simulink model "SF018A_EotProtn"  (R2013b)
settings: Solver=FixedStepDiscrete  SolverMode=SingleTasking  StartTime=0.0  StopTime=0.002  FixedStep=.002  RelTol=1e-3
undefined symbols (not defined in the file): ALLSPDDAMPG_CNT_U08, ALLSPDGAIN_CNT_U08, ARCHGLBPRM_2MILLISEC_SEC_F32, DISTLPFILFRQ_HZ_F32, EOTDAMPGLOLIM_MOTNWTMTR_F32, EOTGAINHILIM_ULS_F32, EotProtnActvRegnBypMaxThd, EotProtnDampgSlew, EotProtnDampgVehSpdTbl, EotProtnDeltaTqThd, EotProtnDftPosn, EotProtnEntrGainVehSpdTbl, EotProtnEntrGainX, EotProtnEntrStLpFilFrq, EotProtnExitDampgY, EotProtnExitStLpFilFrq, EotProtnHwAgGain, EotProtnHwAgMax, EotProtnHwAgMin, EotProtnHwDegDampgX, EotProtnMotSpdIncptSca, EotProtnMotSpdIncptX, EotProtnMotSpdIncptY, EotProtnMotVelGain, EotProtnNormDampgY, EotProtnPosnRampStep, EotProtnRackTrvlLimrAuthyThd, EotProtnRackTrvlLimrAuthyThdLimd, EotProtnRackTrvlLimrEna, EotProtnRackTrvlLimrRng, EotProtnRackTrvlLimrRngLimd, EotProtnRackTrvlLimrVehSpdThd, EotProtnRunEotVelImpctAndSoftEndStop, EotProtnSoftEndStopAuthyThd, EotProtnSoftEndStopEna, EotProtnSoftEndStopVehSpdThd, FIRSTPTDAMPG_CNT_U08, LASTPTGAIN_CNT_U08, SOFTENDSTOPSTDI_CNT_U08, SOFTENDSTOPSTENTR_CNT_U08, SOFTENDSTOPSTEXIT_CNT_U08, SOFTENDSTOPSTNORM_CNT_U08, SYSGLBPRM_MOTTQCMDHILIM_MOTNWTMTR_F32, ZEROMOTTQCMD_MOTNWTMTR_F32
libraries: NxtrAbslt x16, FloatToFixd x14, FixdToFloat x6, Fil x5, NxtrLim x5, simulink x4, NxtrMax x4, LnrIntrpnDyn x3, NxtrSign x2, BilnrIntrpnMplXDyn x2, BilnrIntrpnMplX x1, LnrIntrpn x1
(part 2 of 5)

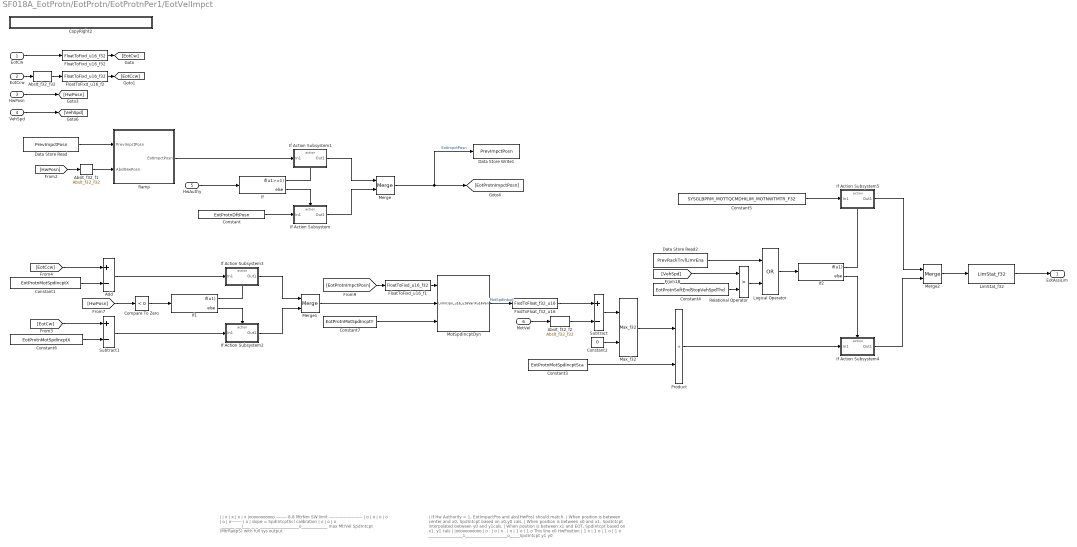
== system SF018A_EotProtn/EotProtn/EotProtnPer1/EotVelImpct ==
  note: |       If Hw Authority = 1, EotImpactPos and abs(HwPos) should match.
      | |        When position is between center and x0, SpdIntcpt based on x0,y0 cals.
      | |        When position is between x0 and x1,        SpdIntcpt interpolated between y0 and y1cals.
      | |        When position is between x1 and EOT,    SpdIntcpt based on x1, y1 cals
      | |
      | |ooooooooooo
      | |                             o                    .
      | |                                   o
      | |                                         o                 .
      | |                                               o
      | | 1                                                  o
      | |       1                                                  o      This line x0 HwPosition
      | |             1                                                  o
      | |                   1                                                  o
      | |                         1                                                  o
      | |                               1                                                  o
      | _________________1_____________________o_____SpdIntcpt
      |                                         y1                                               y0
  note: |
      | | x
      | |       x
      | |             x
      | |                   x
      | |ooooooooooo -------- 8.8 MtrNm SW limit  -------------------------
      | |                             o
      | |                                   o
      | |                                         o
      | |                                               o
      | |                                                     o
      | |                                                           o--------
      | |                                                                 o    |  slope = SpdIntcptScl calibration
      | |                                                                       o
      | |                                                                             o
      | |                                                                                    o
      | ___________|____________________________o_____________
      |                    max MtrVel                                              SpdIntcpt (MtrRadpS)
      |              with full sys output
  EotCw : Inport
  EotCcw : Inport  Port=2
  HwPosn : Inport  Port=3
  VehSpd : Inport  Port=4
  HwAuthy : Inport  Port=5
  MotVel : Inport  Port=6
  Abslt_f32_f1 : NxtrAbslt/Abslt_f32_f32  SFunctionSpec=single y1 = Abslt_f32_f32(single u1)
      settings: AttributesFormatString=%<Name>
  Abslt_f32_f2 : NxtrAbslt/Abslt_f32_f32  SFunctionSpec=single y1 = Abslt_f32_f32(single u1)
      settings: AttributesFormatString=%<Name>
  Abslt_f32_f32 : NxtrAbslt/Abslt_f32_f32  SFunctionSpec=single y1 = Abslt_f32_f32(single u1)
      settings: AttributesFormatString=%<Name>
  Add : Sum  RequirementInfo={'linktype_rmi_doors' '0000ba56 (/E-STEER Core/SubSystem Specifications/Application Functions/SF018A End-of-Travel Actuator Management- EOT Impact and Soft Stops)' '#SF018A_100' 'true' 'REQ: SF018A_100' '' } %GIDa_0ea60b4c_3e02_4ee0_9774_7498ba84a055  Inputs=+-
  Compare To Zero : simulink/Logic and Bit Operations/Compare To Zero  RequirementInfo={'linktype_rmi_doors' '0000ba56 (/E-STEER Core/SubSystem Specifications/Application Functions/SF018A End-of-Travel Actuator Management- EOT Impact and Soft Stops)' '#SF018A_100' 'true' 'REQ: SF018A_100' '' } %GIDa_b6edef5f_67dd_4786_86e6_5c0c809eaf56  relop=<  OutDataTypeStr=boolean
  Constant : Constant  Value=EotProtnDftPosn
  Constant1 : Constant  RequirementInfo={'linktype_rmi_doors' '0000ba56 (/E-STEER Core/SubSystem Specifications/Application Functions/SF018A End-of-Travel Actuator Management- EOT Impact and Soft Stops)' '#SF018A_100' 'true' 'REQ: SF018A_100' '' } %GIDa_8d001312_3515_4819_8386_aa5828f5792f  Value=EotProtnMotSpdIncptX
  Constant2 : Constant  Value=0  OutDataTypeStr=single
  Constant3 : Constant  RequirementInfo={'linktype_rmi_doors' '0000ba56 (/E-STEER Core/SubSystem Specifications/Application Functions/SF018A End-of-Travel Actuator Management- EOT Impact and Soft Stops)' '#SF018A_100' 'true' 'REQ: SF018A_100' '' } %GIDa_e32a7a1c_1bb3_4a5f_bc47_25ead6a9dd83  Value=EotProtnMotSpdIncptSca
  Constant4 : Constant  RequirementInfo={'linktype_rmi_doors' '0000ba56 (/E-STEER Core/SubSystem Specifications/Application Functions/SF018A End-of-Travel Actuator Management- EOT Impact and Soft Stops)' '#SF018A_103' 'true' 'REQ: SF018A_103' '' ; 'linktype_rmi_doors' '0000ba56 (/E-STEER Core/SubSystem Specifications/Application Functions/SF018A End-of-Travel Actuator Management- EOT Impact and Soft Stops)' '#SF018A_101' 'true' 'REQ: SF018A_101' '' } %GIDa_93809a0b_5c17_4f32_b74b_acde70dfea64  Value=EotProtnSoftEndStopVehSpdThd
  Constant5 : Constant  RequirementInfo={'linktype_rmi_doors' '0000ba56 (/E-STEER Core/SubSystem Specifications/Application Functions/SF018A End-of-Travel Actuator Management- EOT Impact and Soft Stops)' '#SF018A_98' 'true' 'REQ: SF018A_98' '' } %GIDa_8f6ebd6e_ac8a_4b56_8ce0_6dc234867ca6  Value=SYSGLBPRM_MOTTQCMDHILIM_MOTNWTMTR_F32
  Constant6 : Constant  RequirementInfo={'linktype_rmi_doors' '0000ba56 (/E-STEER Core/SubSystem Specifications/Application Functions/SF018A End-of-Travel Actuator Management- EOT Impact and Soft Stops)' '#SF018A_100' 'true' 'REQ: SF018A_100' '' } %GIDa_e8e2a964_e133_4f7b_9159_11a485f41865  Value=EotProtnMotSpdIncptX
  Constant7 : Constant  RequirementInfo={'linktype_rmi_doors' '0000ba56 (/E-STEER Core/SubSystem Specifications/Application Functions/SF018A End-of-Travel Actuator Management- EOT Impact and Soft Stops)' '#SF018A_100' 'true' 'REQ: SF018A_100' '' } %GIDa_e0aa8e23_046e_4471_9def_99ca72f23587  Value=EotProtnMotSpdIncptY
  CopyRight2 : Subsystem  Description=|  mask(Copyright Information){none=on}
      | Copyright info block.                                               
      |                                                                     
      | Place copyright information at the top of every subsystem in design.
      mask prompts: none "No parameters"
      mask help: Place copyright information at the top of every subsystem in design.
      mask Display:
      | NxtrConf = 'Nexteer Confidential';
      | 
      | sys = bdroot; %handle for the current model ("system")
      | first = get_param(sys,'Created');
      | if(isempty(first))
      |     first = datestr(now,'yyyy');
      | else
      |     first = first(end-3:end);  %year is last four digits
      | end
      | 
      | last = get_param(sys,'LastModifiedDate');
      | if isempty(last)
      |     last = datestr(now,'yyyy');
      | else
      |     last = last(end-3:end);
      | end
      | 
      | if strcmp(first,last)
      |     fprintf('%s -- Copyright %s Nexteer',NxtrConf,first)
      | else
      |     fprintf('%s -- %s%s- %s Nexteer',NxtrConf,char(169),first,last)
      | end
  Data Store Read : DataStoreRead  DataStoreName=PrevImpctPosn
  Data Store Read2 : DataStoreRead  RequirementInfo={'linktype_rmi_doors' '0000ba56 (/E-STEER Core/SubSystem Specifications/Application Functions/SF018A End-of-Travel Actuator Management- EOT Impact and Soft Stops)' '#SF018A_103' 'true' 'REQ: SF018A_103' '' ; 'linktype_rmi_doors' '0000ba56 (/E-STEER Core/SubSystem Specifications/Application Functions/SF018A End-of-Travel Actuator Management- EOT Impact and Soft Stops)' '#SF018A_101' 'true' 'REQ: SF018A_101' '' } %GIDa_5d85e818_9e51_4cc9_980e_2c33546dc9c1  DataStoreName=PrevRackTrvlLimrEna
  Data Store Write1 : DataStoreWrite  DataStoreName=PrevImpctPosn
  FixdToFloat_f32_u16 : FixdToFloat/FixdToFloat_f32_u16  Param1=4
  FloatToFixd_u16_f1 : FloatToFixd/FloatToFixd_u16_f32  Param1=4
  FloatToFixd_u16_f2 : FloatToFixd/FloatToFixd_u16_f32  Param1=4
  FloatToFixd_u16_f32 : FloatToFixd/FloatToFixd_u16_f32  Param1=4
  If : If  RequirementInfo={'linktype_rmi_doors' '0000ba56 (/E-STEER Core/SubSystem Specifications/Application Functions/SF018A End-of-Travel Actuator Management- EOT Impact and Soft Stops)' '#SF018A_99' 'true' 'REQ: SF018A_99' '' } %GIDa_114076bb_8725_4b92_80f1_73db1f525c76  IfExpression=u1>=1
  If Action Subsystem : Subsystem  RequirementInfo={'linktype_rmi_doors' '0000ba56 (/E-STEER Core/SubSystem Specifications/Application Functions/SF018A End-of-Travel Actuator Management- EOT Impact and Soft Stops)' '#SF018A_99' 'true' 'REQ: SF018A_99' '' } %GIDa_616af379_9c94_4833_8ebd_97394973f79f  TreatAsAtomicUnit=on
  If Action Subsystem1 : Subsystem  RequirementInfo={'linktype_rmi_doors' '0000ba56 (/E-STEER Core/SubSystem Specifications/Application Functions/SF018A End-of-Travel Actuator Management- EOT Impact and Soft Stops)' '#SF018A_99' 'true' 'REQ: SF018A_99' '' } %GIDa_2c9b4916_e802_4e25_825d_e1601ce296ae  TreatAsAtomicUnit=on
  If Action Subsystem2 : Subsystem  RequirementInfo={'linktype_rmi_doors' '0000ba56 (/E-STEER Core/SubSystem Specifications/Application Functions/SF018A End-of-Travel Actuator Management- EOT Impact and Soft Stops)' '#SF018A_100' 'true' 'REQ: SF018A_100' '' } %GIDa_9326fc4b_b234_4fd5_839c_5948232246f9  TreatAsAtomicUnit=on
  If Action Subsystem3 : Subsystem  RequirementInfo={'linktype_rmi_doors' '0000ba56 (/E-STEER Core/SubSystem Specifications/Application Functions/SF018A End-of-Travel Actuator Management- EOT Impact and Soft Stops)' '#SF018A_100' 'true' 'REQ: SF018A_100' '' } %GIDa_5a238f3e_6544_4bb4_b8fd_4b11bcca8e10  TreatAsAtomicUnit=on
  If Action Subsystem4 : Subsystem  RequirementInfo={'linktype_rmi_doors' '0000ba56 (/E-STEER Core/SubSystem Specifications/Application Functions/SF018A End-of-Travel Actuator Management- EOT Impact and Soft Stops)' '#SF018A_98' 'true' 'REQ: SF018A_98' '' } %GIDa_ee8eac1b_f706_4a22_9467_09c0bfa4fe0d  TreatAsAtomicUnit=on
  If Action Subsystem5 : Subsystem  RequirementInfo={'linktype_rmi_doors' '0000ba56 (/E-STEER Core/SubSystem Specifications/Application Functions/SF018A End-of-Travel Actuator Management- EOT Impact and Soft Stops)' '#SF018A_98' 'true' 'REQ: SF018A_98' '' } %GIDa_87c38652_44bd_4824_bc16_f0213d33fe08  TreatAsAtomicUnit=on
  If1 : If  RequirementInfo={'linktype_rmi_doors' '0000ba56 (/E-STEER Core/SubSystem Specifications/Application Functions/SF018A End-of-Travel Actuator Management- EOT Impact and Soft Stops)' '#SF018A_100' 'true' 'REQ: SF018A_100' '' } %GIDa_01c461cb_08e0_4434_9ddb_fa4f29abf7ef  IfExpression=u1
  If2 : If  RequirementInfo={'linktype_rmi_doors' '0000ba56 (/E-STEER Core/SubSystem Specifications/Application Functions/SF018A End-of-Travel Actuator Management- EOT Impact and Soft Stops)' '#SF018A_98' 'true' 'REQ: SF018A_98' '' } %GIDa_08a42b5d_cfca_463b_971f_377684ad0b46  IfExpression=u1
  LimStat_f32 : NxtrLim/LimStat_f32  RequirementInfo={'linktype_rmi_doors' '0000ba56 (/E-STEER Core/SubSystem Specifications/Application Functions/SF018A End-of-Travel Actuator Management- EOT Impact and Soft Stops)' '#SF018A_98' 'true' 'REQ: SF018A_98' '' } %GIDa_7d65fa4b_23cc_4559_9257_d752ae61080a  LoLim=ZEROMOTTQCMD_MOTNWTMTR_F32  HiLim=SYSGLBPRM_MOTTQCMDHILIM_MOTNWTMTR_F32
      settings: AttributesFormatString=|
      | Low Limit: %<LoLim>
      | High Limit:%<HiLim>
  Logical Operator : Logic  RequirementInfo={'linktype_rmi_doors' '0000ba56 (/E-STEER Core/SubSystem Specifications/Application Functions/SF018A End-of-Travel Actuator Management- EOT Impact and Soft Stops)' '#SF018A_101' 'true' 'REQ: SF018A_101' '' ; 'linktype_rmi_doors' '0000ba56 (/E-STEER Core/SubSystem Specifications/Application Functions/SF018A End-of-Travel Actuator Management- EOT Impact and Soft Stops)' '#SF018A_103' 'true' 'REQ: SF018A_103' '' } %GIDa_ff2f1a2c_ffd8_4347_a43f_f58ee380b49f  Operator=OR  AllPortsSameDT=off  OutDataTypeStr=boolean
  Max_f32 : NxtrMax/Max_f32  SFunctionSpec=single y1 = Max_f32(single u1, single u2)
      settings: AttributesFormatString=%<Name>
  Merge : Merge  RequirementInfo={'linktype_rmi_doors' '0000ba56 (/E-STEER Core/SubSystem Specifications/Application Functions/SF018A End-of-Travel Actuator Management- EOT Impact and Soft Stops)' '#SF018A_99' 'true' 'REQ: SF018A_99' '' } %GIDa_3ccaa3b7_e9a6_4bd2_b01b_e13117ad3d2a
  Merge1 : Merge  RequirementInfo={'linktype_rmi_doors' '0000ba56 (/E-STEER Core/SubSystem Specifications/Application Functions/SF018A End-of-Travel Actuator Management- EOT Impact and Soft Stops)' '#SF018A_100' 'true' 'REQ: SF018A_100' '' } %GIDa_4508a611_5f6d_4e15_8a69_017cc3ebf3d9
  Merge2 : Merge  RequirementInfo={'linktype_rmi_doors' '0000ba56 (/E-STEER Core/SubSystem Specifications/Application Functions/SF018A End-of-Travel Actuator Management- EOT Impact and Soft Stops)' '#SF018A_98' 'true' 'REQ: SF018A_98' '' } %GIDa_c2d7a1d8_9443_4fb2_b4b1_13f2c12ecdc5
  MotSpdIncptDyn : LnrIntrpnDyn/LnrIntrpn_u16_u16VariXu16VariY  RequirementInfo={'linktype_rmi_doors' '0000ba56 (/E-STEER Core/SubSystem Specifications/Application Functions/SF018A End-of-Travel Actuator Management- EOT Impact and Soft Stops)' '#SF018A_100' 'true' 'REQ: SF018A_100' '' ; 'linktype_rmi_doors' '0000ba56 (/E-STEER Core/SubSystem Specifications/Application Functions/SF018A End-of-Travel Actuator Management- EOT Impact and Soft Stops)' '#SF018A_99' 'true' 'REQ: SF018A_99' '' } %GIDa_feb0f20b_0c88_497f_9d91_df13f9652457
      settings: AttributesFormatString=Lnr ( u16VariX , u16VariY )
  Product : Product  RequirementInfo={'linktype_rmi_doors' '0000ba56 (/E-STEER Core/SubSystem Specifications/Application Functions/SF018A End-of-Travel Actuator Management- EOT Impact and Soft Stops)' '#SF018A_100' 'true' 'REQ: SF018A_100' '' } %GIDa_dd6beda9_3314_4949_8896_a1bfb102cc0b  RndMeth=Zero
  Ramp : Subsystem  RequirementInfo={'linktype_rmi_doors' '0000ba56 (/E-STEER Core/SubSystem Specifications/Application Functions/SF018A End-of-Travel Actuator Management- EOT Impact and Soft Stops)' '#SF018A_99' 'true' 'REQ: SF018A_99' '' } %GIDa_506432ef_6bac_4bcd_b546_3f821148aaf5
  Relational Operator : RelationalOperator  RequirementInfo={'linktype_rmi_doors' '0000ba56 (/E-STEER Core/SubSystem Specifications/Application Functions/SF018A End-of-Travel Actuator Management- EOT Impact and Soft Stops)' '#SF018A_103' 'true' 'REQ: SF018A_103' '' ; 'linktype_rmi_doors' '0000ba56 (/E-STEER Core/SubSystem Specifications/Application Functions/SF018A End-of-Travel Actuator Management- EOT Impact and Soft Stops)' '#SF018A_101' 'true' 'REQ: SF018A_101' '' } %GIDa_17e498e1_13fa_4fd0_801a_ca4bfebf577c  Operator=>  OutDataTypeStr=boolean
  Subtract : Sum  RequirementInfo={'linktype_rmi_doors' '0000ba56 (/E-STEER Core/SubSystem Specifications/Application Functions/SF018A End-of-Travel Actuator Management- EOT Impact and Soft Stops)' '#SF018A_99' 'true' 'REQ: SF018A_99' '' ; 'linktype_rmi_doors' '0000ba56 (/E-STEER Core/SubSystem Specifications/Application Functions/SF018A End-of-Travel Actuator Management- EOT Impact and Soft Stops)' '#SF018A_100' 'true' 'REQ: SF018A_100' '' } %GIDa_74ee266a_b85a_4dbe_8dec_9fc08d52fda3  Inputs=+-
  Subtract1 : Sum  RequirementInfo={'linktype_rmi_doors' '0000ba56 (/E-STEER Core/SubSystem Specifications/Application Functions/SF018A End-of-Travel Actuator Management- EOT Impact and Soft Stops)' '#SF018A_100' 'true' 'REQ: SF018A_100' '' } %GIDa_3403adc0_af84_4072_930d_8fe9dc0520d9  Inputs=+-
  EotAssiLim : Outport
  wires:
  Constant7/1 -> MotSpdIncptDyn/3
  Merge1/1 -> MotSpdIncptDyn/2
  Subtract1/1 -> If Action Subsystem2/1(In1)
  Abslt_f32_f2/1 -> Subtract/2
  Add/1 -> If Action Subsystem3/1(In1)
  Constant1/1 -> Add/2
  LimStat_f32/1 -> EotAssiLim/1
  Constant3/1 -> Product/2
  Max_f32/1 -> Product/1
  FloatToFixd_u16_f1/1 -> MotSpdIncptDyn/1
  FixdToFloat_f32_u16/1 -> Subtract/1
  MotSpdIncptDyn/1 -> FixdToFloat_f32_u16/1  "MotSpdIntcpt"
  Constant2/1 -> Max_f32/2
  Subtract/1 -> Max_f32/1
  MotVel/1 -> Abslt_f32_f2/1
  FloatToFixd_u16_f32/1 -> [EotCw]
  FloatToFixd_u16_f2/1 -> [EotCcw]
  [EotCw] -> Subtract1/1
  [EotCcw] -> Add/1
  If1/1 -> If Action Subsystem3/Action
  If1/2 -> If Action Subsystem2/Action
  If Action Subsystem2/1(Out1) -> Merge1/2
  If Action Subsystem3/1(Out1) -> Merge1/1
  Constant6/1 -> Subtract1/2
  [EotProtnImpctPosn] -> FloatToFixd_u16_f1/1
  [HwPosn] -> Compare To Zero/1
  Compare To Zero/1 -> If1/1
  Merge/1 -> Data Store Write1/1, [EotProtnImpctPosn]  "EotImpctPosn"
  Constant/1 -> If Action Subsystem/1(In1)
  If/1 -> If Action Subsystem1/Action
  If/2 -> If Action Subsystem/Action
  If Action Subsystem/1(Out1) -> Merge/2
  If Action Subsystem1/1(Out1) -> Merge/1
  Ramp/1(EotImpctPosn) -> If Action Subsystem1/1(In1)
  HwAuthy/1 -> If/1
  Abslt_f32_f1/1 -> Ramp/2(AbsltHwPosn)
  Data Store Read/1 -> Ramp/1(PrevImpctPosn)
  [HwPosn] -> Abslt_f32_f1/1
  VehSpd/1 -> [VehSpd]
  HwPosn/1 -> [HwPosn]
  EotCcw/1 -> Abslt_f32_f32/1
  EotCw/1 -> FloatToFixd_u16_f32/1
  Abslt_f32_f32/1 -> FloatToFixd_u16_f2/1
  [VehSpd] -> Relational Operator/1
  Constant4/1 -> Relational Operator/2
  Relational Operator/1 -> Logical Operator/2
  Data Store Read2/1 -> Logical Operator/1
  Product/1 -> If Action Subsystem4/1(In1)
  If Action Subsystem5/1(Out1) -> Merge2/1
  If2/2 -> If Action Subsystem4/Action
  If2/1 -> If Action Subsystem5/Action
  If Action Subsystem4/1(Out1) -> Merge2/2
  Logical Operator/1 -> If2/1
  Constant5/1 -> If Action Subsystem5/1(In1)
  Merge2/1 -> LimStat_f32/1

== system SF018A_EotProtn/EotProtn/EotProtnPer1/If Action Subsystem ==
  In1 : Inport
  Action Port : ActionPort  ActionType=else
  CopyRight2 : Subsystem  Description=|  mask(Copyright Information){none=on}
      | Copyright info block.                                               
      |                                                                     
      | Place copyright information at the top of every subsystem in design.
      mask prompts: none "No parameters"
      mask help: Place copyright information at the top of every subsystem in design.
      mask Display:
      | NxtrConf = 'Nexteer Confidential';
      | 
      | sys = bdroot; %handle for the current model ("system")
      | first = get_param(sys,'Created');
      | if(isempty(first))
      |     first = datestr(now,'yyyy');
      | else
      |     first = first(end-3:end);  %year is last four digits
      | end
      | 
      | last = get_param(sys,'LastModifiedDate');
      | if isempty(last)
      |     last = datestr(now,'yyyy');
      | else
      |     last = last(end-3:end);
      | end
      | 
      | if strcmp(first,last)
      |     fprintf('%s -- Copyright %s Nexteer',NxtrConf,first)
      | else
      |     fprintf('%s -- %s%s- %s Nexteer',NxtrConf,char(169),first,last)
      | end
  Out1 : Outport
  wires:
  In1/1 -> Out1/1

== system SF018A_EotProtn/EotProtn/EotProtnPer1/If Action Subsystem5 ==
  In1 : Inport
  Action Port : ActionPort  ActionType=then
  CopyRight2 : Subsystem  Description=|  mask(Copyright Information){none=on}
      | Copyright info block.                                               
      |                                                                     
      | Place copyright information at the top of every subsystem in design.
      mask prompts: none "No parameters"
      mask help: Place copyright information at the top of every subsystem in design.
      mask Display:
      | NxtrConf = 'Nexteer Confidential';
      | 
      | sys = bdroot; %handle for the current model ("system")
      | first = get_param(sys,'Created');
      | if(isempty(first))
      |     first = datestr(now,'yyyy');
      | else
      |     first = first(end-3:end);  %year is last four digits
      | end
      | 
      | last = get_param(sys,'LastModifiedDate');
      | if isempty(last)
      |     last = datestr(now,'yyyy');
      | else
      |     last = last(end-3:end);
      | end
      | 
      | if strcmp(first,last)
      |     fprintf('%s -- Copyright %s Nexteer',NxtrConf,first)
      | else
      |     fprintf('%s -- %s%s- %s Nexteer',NxtrConf,char(169),first,last)
      | end
  Out1 : Outport
  wires:
  In1/1 -> Out1/1

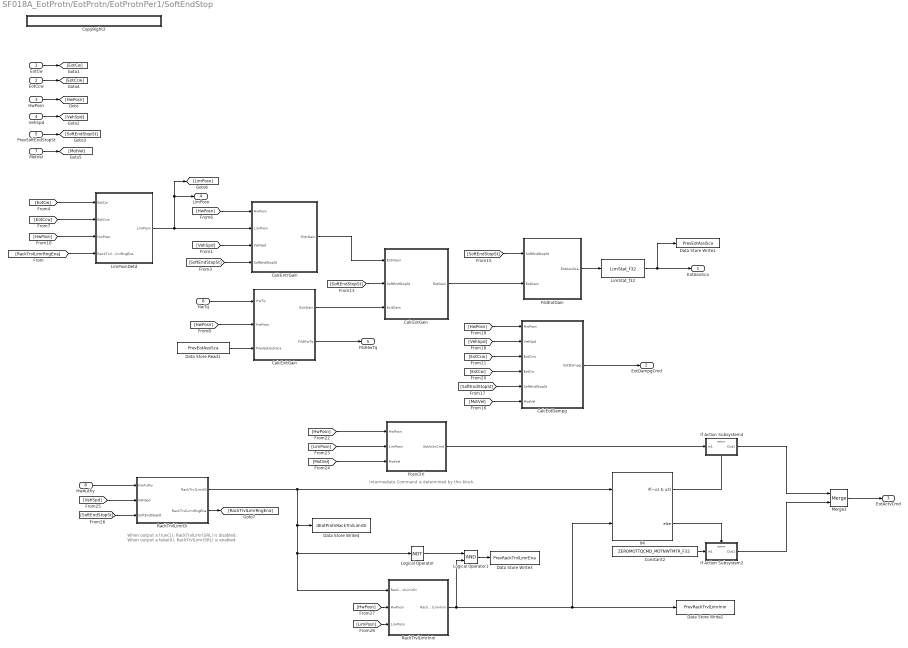
== system SF018A_EotProtn/EotProtn/EotProtnPer1/SoftEndStop ==
  note: When output a true(1), RackTrvlLimr(SRL) is disabled;
      | When output a false(0), RackTrvlLimr(SRL) is enabled.
  note: Intermediate Command is determined by this block.
  EotCw : Inport
  EotCcw : Inport  Port=2
  HwPosn : Inport  Port=3
  VehSpd : Inport  Port=4
  PrevSoftEndStopSt : Inport  Port=5
  HwTq : Inport  Port=6
  MotVel : Inport  Port=7
  HwAuthy : Inport  Port=8
  CalcEntrGain : Subsystem
  CalcEotDampg : Subsystem
  CalcEotGain : Subsystem
  CalcExitGain : Subsystem
  Constant2 : Constant  RequirementInfo={'linktype_rmi_doors' '0000ba56 (/E-STEER Core/SubSystem Specifications/Application Functions/SF018A End-of-Travel Actuator Management- EOT Impact and Soft Stops)' '#SF018A_123' 'true' 'REQ: SF018A_123' '' } %GIDa_ca75b6e7_9b62_43a2_9e72_9f9cd1615950  Value=ZEROMOTTQCMD_MOTNWTMTR_F32
  CopyRight2 : Subsystem  Description=|  mask(Copyright Information){none=on}
      | Copyright info block.                                               
      |                                                                     
      | Place copyright information at the top of every subsystem in design.
      mask prompts: none "No parameters"
      mask help: Place copyright information at the top of every subsystem in design.
      mask Display:
      | NxtrConf = 'Nexteer Confidential';
      | 
      | sys = bdroot; %handle for the current model ("system")
      | first = get_param(sys,'Created');
      | if(isempty(first))
      |     first = datestr(now,'yyyy');
      | else
      |     first = first(end-3:end);  %year is last four digits
      | end
      | 
      | last = get_param(sys,'LastModifiedDate');
      | if isempty(last)
      |     last = datestr(now,'yyyy');
      | else
      |     last = last(end-3:end);
      | end
      | 
      | if strcmp(first,last)
      |     fprintf('%s -- Copyright %s Nexteer',NxtrConf,first)
      | else
      |     fprintf('%s -- %s%s- %s Nexteer',NxtrConf,char(169),first,last)
      | end
  Data Store Read1 : DataStoreRead  DataStoreName=PrevEotAssiSca
  Data Store Write1 : DataStoreWrite  DataStoreName=PrevEotAssiSca
  Data Store Write2 : DataStoreWrite  RequirementInfo={} %GIDa_96f80f9a_e8fa_4104_938d_35aeb3800faa  DataStoreName=PrevRackTrvlLimrInin
  Data Store Write3 : DataStoreWrite  DataStoreName=PrevRackTrvlLimrEna
  Data Store Write4 : DataStoreWrite  DataStoreName=dEotProtnRackTrvlLimrDi
  FildEotGain : Subsystem
  If Action Subsystem2 : Subsystem  RequirementInfo={'linktype_rmi_doors' '0000ba56 (/E-STEER Core/SubSystem Specifications/Application Functions/SF018A End-of-Travel Actuator Management- EOT Impact and Soft Stops)' '#SF018A_123' 'true' 'REQ: SF018A_123' '' } %GIDa_60d4082f_db6f_4d15_9780_0544a011027c  TreatAsAtomicUnit=on
  If Action Subsystem4 : Subsystem  RequirementInfo={'linktype_rmi_doors' '0000ba56 (/E-STEER Core/SubSystem Specifications/Application Functions/SF018A End-of-Travel Actuator Management- EOT Impact and Soft Stops)' '#SF018A_123' 'true' 'REQ: SF018A_123' '' } %GIDa_ae86effe_7463_494a_8592_ff26dad16a83  TreatAsAtomicUnit=on
  If4 : If  RequirementInfo={'linktype_rmi_doors' '0000ba56 (/E-STEER Core/SubSystem Specifications/Application Functions/SF018A End-of-Travel Actuator Management- EOT Impact and Soft Stops)' '#SF018A_123' 'true' 'REQ: SF018A_123' '' } %GIDa_b79cbd39_9320_4638_a12a_0906b0122338  NumInputs=2  IfExpression=~u1 & u2
  LimPosnDetd : Subsystem
  LimStat_f32 : NxtrLim/LimStat_f32  RequirementInfo={'linktype_rmi_doors' '0000ba56 (/E-STEER Core/SubSystem Specifications/Application Functions/SF018A End-of-Travel Actuator Management- EOT Impact and Soft Stops)' '#SF018A_106' 'true' 'REQ: SF018A_106' '' ; 'linktype_rmi_doors' '0000ba56 (/E-STEER Core/SubSystem Specifications/Application Functions/SF018A End-of-Travel Actuator Management- EOT Impact and Soft Stops)' '#SF018A_109' 'true' 'REQ: SF018A_109' '' } %GIDa_775b1e77_290a_4b22_93c1_34ff83087529  LoLim=EOTGAINLOLIM_ULS_F32  HiLim=EOTGAINHILIM_ULS_F32
      settings: AttributesFormatString=|
      | Low Limit: %<LoLim>
      | High Limit:%<HiLim>
  Logical Operator : Logic  Operator=NOT  AllPortsSameDT=off  OutDataTypeStr=boolean
  Logical Operator1 : Logic  AllPortsSameDT=off  OutDataTypeStr=boolean
  Merge3 : Merge  RequirementInfo={'linktype_rmi_doors' '0000ba56 (/E-STEER Core/SubSystem Specifications/Application Functions/SF018A End-of-Travel Actuator Management- EOT Impact and Soft Stops)' '#SF018A_123' 'true' 'REQ: SF018A_123' '' } %GIDa_9578766e_a356_41cb_bf87_d13ebc1589a4
  PosnCtrl : Subsystem
  RackTrvlLimrDi : Subsystem
  RackTrvlLimrInin : Subsystem
  EotAssiSca : Outport
  EotDampgCmd : Outport  Port=2
  EotActvCmd : Outport  Port=3
  LimPosn : Outport  Port=4
  FildHwTq : Outport  Port=5
  wires:
  PosnCtrl/1(EotActvCmd) -> If Action Subsystem4/1(In1)
  Logical Operator1/1 -> Data Store Write3/1
  Logical Operator/1 -> Logical Operator1/1
  RackTrvlLimrDi/1(RackTrvlLimrDi) -> RackTrvlLimrInin/1(RackTrvlLimrDi), Logical Operator/1, Data Store Write4/1, If4/1
  [LimPosn] -> RackTrvlLimrInin/3(LimPosn)
  [HwPosn] -> RackTrvlLimrInin/2(HwPosn)
  RackTrvlLimrInin/1(RackTrvlLimrInin) -> If4/2, Data Store Write2/1, Logical Operator1/2
  [SoftEndStopSt] -> RackTrvlLimrDi/3(SoftEndStopSt)
  [VehSpd] -> RackTrvlLimrDi/2(VehSpd)
  HwAuthy/1 -> RackTrvlLimrDi/1(HwAuthy)
  Merge3/1 -> EotActvCmd/1
  If Action Subsystem2/1(Out1) -> Merge3/2
  If Action Subsystem4/1(Out1) -> Merge3/1
  If4/1 -> If Action Subsystem4/Action
  [MotVel] -> PosnCtrl/3(MotVel)
  [LimPosn] -> PosnCtrl/2(LimPosn)
  [HwPosn] -> PosnCtrl/1(HwPosn)
  [EotCcw] -> CalcEotDampg/3(EotCcw)
  [EotCw] -> CalcEotDampg/4(EotCw)
  [HwPosn] -> CalcEotDampg/1(HwPosn)
  [VehSpd] -> CalcEotDampg/2(VehSpd)
  [SoftEndStopSt] -> CalcEotDampg/5(SoftEndStopSt)
  [MotVel] -> CalcEotDampg/6(MotVel)
  MotVel/1 -> [MotVel]
  CalcEotDampg/1(EotDampg) -> EotDampgCmd/1
  [SoftEndStopSt] -> FildEotGain/1(SoftEndStopSt)
  CalcEotGain/1(EotGain) -> FildEotGain/2(EotGain)
  [SoftEndStopSt] -> CalcEotGain/2(SoftEndStopSt)
  CalcExitGain/2(FildHwTq) -> FildHwTq/1
  CalcExitGain/1(ExitGain) -> CalcEotGain/3(ExitGain)
  CalcEntrGain/1(EntrGain) -> CalcEotGain/1(EntrGain)
  Data Store Read1/1 -> CalcExitGain/3(PrevEotAssiSca)
  [HwPosn] -> CalcExitGain/2(HwPosn)
  HwTq/1 -> CalcExitGain/1(HwTq)
  [HwPosn] -> CalcEntrGain/1(HwPosn)
  [SoftEndStopSt] -> CalcEntrGain/4(SoftEndStopSt)
  [VehSpd] -> CalcEntrGain/3(VehSpd)
  [HwPosn] -> LimPosnDetd/3(HwPosn)
  [EotCcw] -> LimPosnDetd/2(EotCcw)
  [EotCw] -> LimPosnDetd/1(EotCw)
  LimPosnDetd/1(LimPosn) -> LimPosn/1, [LimPosn], CalcEntrGain/2(LimPosn)
  PrevSoftEndStopSt/1 -> [SoftEndStopSt]
  VehSpd/1 -> [VehSpd]
  EotCcw/1 -> [EotCcw]
  EotCw/1 -> [EotCw]
  HwPosn/1 -> [HwPosn]
  FildEotGain/1(EotAssiSca) -> LimStat_f32/1
  LimStat_f32/1 -> EotAssiSca/1, Data Store Write1/1
  Constant2/1 -> If Action Subsystem2/1(In1)
  If4/2 -> If Action Subsystem2/Action
  RackTrvlLimrDi/2(RackTrvlLimrRngEna) -> [RackTrvlLimrRngEna]
  [RackTrvlLimrRngEna] -> LimPosnDetd/4(RackTrvlLimrRngEna)

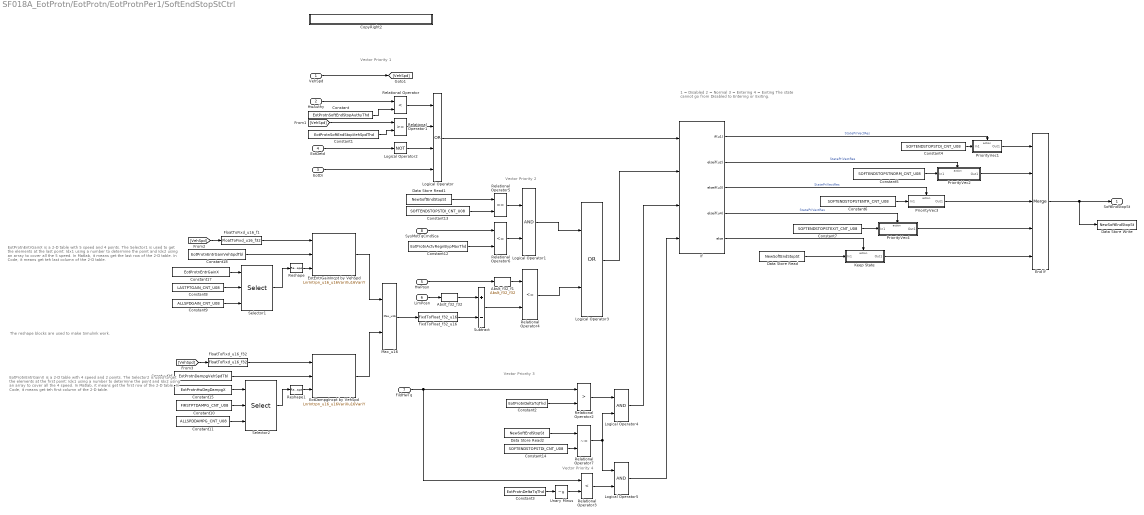
== system SF018A_EotProtn/EotProtn/EotProtnPer1/SoftEndStopStCtrl ==
  note: EotProtnEntrGainX is a 2-D table with 4 speed and 2 points.  The Selector2 is used to
      | get the elements at the first point: Idx1 using a number to determine the point and Idx2
      | using an array to cover all the 4 speed.
      |
      | In Matlab, it means get the first row of the 2-D table.
      | In Code, it means get teh first column of the 2-D table.
  note: EotProtnEntrGainX is a 2-D table with 5 speed and 4 points.  The Selector1 is used to
      | get the elements at the last point: Idx1 using a number to determine the point and Idx2
      | using an array to cover all the 5 speed.
      |
      | In Matlab,  it means get the last row of the 2-D table.
      | In Code, it means get teh last column of the 2-D table.
  note: Vector Priority 4
  note: Vector Priority 2
  note: Vector Priority 1
  note: 1 = Disabled
      | 2 = Normal
      | 3 = Entering
      | 4 = Exiting
      |
      | The state cannot go from Disabled to Entering or Exiting.
  note: Vector Priority 3
  note: The reshape blocks are used to make Simulink work.
  VehSpd : Inport
  HwAuthy : Inport  Port=2
  EotDi : Inport  Port=3
  EotDetd : Inport  Port=4
  HwPosn : Inport  Port=5
  LimPosn : Inport  Port=6
  FildHwTq : Inport  Port=7
  SysMotTqCmdSca : Inport  Port=8
  Abslt_f32_f1 : NxtrAbslt/Abslt_f32_f32  SFunctionSpec=single y1 = Abslt_f32_f32(single u1)
      settings: AttributesFormatString=%<Name>
  Abslt_f32_f32 : NxtrAbslt/Abslt_f32_f32  SFunctionSpec=single y1 = Abslt_f32_f32(single u1)
      settings: AttributesFormatString=%<Name>
  Constant : Constant  Value=EotProtnSoftEndStopAuthyThd
  Constant1 : Constant  Value=EotProtnSoftEndStopVehSpdThd
  Constant10 : Constant  Value=FIRSTPTDAMPG_CNT_U08
  Constant11 : Constant  Value=ALLSPDDAMPG_CNT_U08
  Constant12 : Constant  Value=EotProtnActvRegnBypMaxThd
  Constant13 : Constant  Value=SOFTENDSTOPSTDI_CNT_U08
  Constant14 : Constant  Value=SOFTENDSTOPSTDI_CNT_U08
  Constant15 : Constant  Value=EotProtnHwDegDampgX
  Constant16 : Constant  Value=EotProtnDampgVehSpdTbl
  Constant17 : Constant  Value=EotProtnEntrGainX
  Constant18 : Constant  Value=EotProtnEntrGainVehSpdTbl
  Constant2 : Constant  Value=EotProtnDeltaTqThd
  Constant3 : Constant  Value=EotProtnDeltaTqThd
  Constant4 : Constant  Value=SOFTENDSTOPSTDI_CNT_U08
  Constant5 : Constant  Value=SOFTENDSTOPSTNORM_CNT_U08
  Constant6 : Constant  Value=SOFTENDSTOPSTENTR_CNT_U08
  Constant7 : Constant  Value=SOFTENDSTOPSTEXIT_CNT_U08
  Constant8 : Constant  Value=LASTPTGAIN_CNT_U08
  Constant9 : Constant  Value=ALLSPDGAIN_CNT_U08
  CopyRight2 : Subsystem  Description=|  mask(Copyright Information){none=on}
      | Copyright info block.                                               
      |                                                                     
      | Place copyright information at the top of every subsystem in design.
      mask prompts: none "No parameters"
      mask help: Place copyright information at the top of every subsystem in design.
      mask Display:
      | NxtrConf = 'Nexteer Confidential';
      | 
      | sys = bdroot; %handle for the current model ("system")
      | first = get_param(sys,'Created');
      | if(isempty(first))
      |     first = datestr(now,'yyyy');
      | else
      |     first = first(end-3:end);  %year is last four digits
      | end
      | 
      | last = get_param(sys,'LastModifiedDate');
      | if isempty(last)
      |     last = datestr(now,'yyyy');
      | else
      |     last = last(end-3:end);
      | end
      | 
      | if strcmp(first,last)
      |     fprintf('%s -- Copyright %s Nexteer',NxtrConf,first)
      | else
      |     fprintf('%s -- %s%s- %s Nexteer',NxtrConf,char(169),first,last)
      | end
  Data Store Read : DataStoreRead  DataStoreName=NewSoftEndStopSt
  Data Store Read1 : DataStoreRead  DataStoreName=NewSoftEndStopSt
  Data Store Read2 : DataStoreRead  DataStoreName=NewSoftEndStopSt
  Data Store Write : DataStoreWrite  DataStoreName=NewSoftEndStopSt
  End If : Merge  Inputs=5
  EotDampgIncpt by VehSpd : LnrIntrpnDyn/LnrIntrpn_u16_u16VariXu16VariY
      settings: AttributesFormatString=Lnr ( u16VariX , u16VariY )
  EotEntrGainIncpt by VehSpd : LnrIntrpnDyn/LnrIntrpn_u16_u16VariXu16VariY
      settings: AttributesFormatString=Lnr ( u16VariX , u16VariY )
  FixdToFloat_f32_u16 : FixdToFloat/FixdToFloat_f32_u16  Param1=4
  FloatToFixd_u16_f1 : FloatToFixd/FloatToFixd_u16_f32  Param1=7
  FloatToFixd_u16_f32 : FloatToFixd/FloatToFixd_u16_f32  Param1=7
  If : If  NumInputs=4  IfExpression=u1  ElseIfExpressions=u2, u3, u4
  Keep State : Subsystem
  Logical Operator : Logic  Operator=OR  Inputs=4  AllPortsSameDT=off  OutDataTypeStr=boolean
  Logical Operator1 : Logic  AllPortsSameDT=off  OutDataTypeStr=boolean
  Logical Operator2 : Logic  Operator=NOT  Inputs=1  AllPortsSameDT=off  OutDataTypeStr=boolean
  Logical Operator3 : Logic  Operator=OR  AllPortsSameDT=off  OutDataTypeStr=boolean
  Logical Operator4 : Logic  AllPortsSameDT=off  OutDataTypeStr=boolean
  Logical Operator5 : Logic  AllPortsSameDT=off  OutDataTypeStr=boolean
  Max_u16 : NxtrMax/Max_u16  SFunctionSpec=uint16 y1 = Max_u16(uint16 u1, uint16 u2)
      settings: AttributesFormatString=%<Name>
  PriorityVec1 : Subsystem
  PriorityVec2 : Subsystem
  PriorityVec3 : Subsystem
  PriorityVec4 : Subsystem
  Relational Operator : RelationalOperator  Operator=<  OutDataTypeStr=boolean
  Relational Operator1 : RelationalOperator  OutDataTypeStr=boolean
  Relational Operator2 : RelationalOperator  Operator=>  OutDataTypeStr=boolean
  Relational Operator3 : RelationalOperator  Operator=<  OutDataTypeStr=boolean
  Relational Operator4 : RelationalOperator  Operator=<=  OutDataTypeStr=boolean
  Relational Operator5 : RelationalOperator  Operator===  OutDataTypeStr=boolean
  Relational Operator6 : RelationalOperator  Operator=<=  OutDataTypeStr=boolean
  Relational Operator7 : RelationalOperator  Operator=~=  OutDataTypeStr=boolean
  Reshape : Reshape
  Reshape1 : Reshape
  Selector1 : Selector  NumberOfDimensions=2  IndexMode=Zero-based  IndexOptions=Index vector (port),Index vector (port)  Indices=3,[0:4]  OutputSizes=1,1
  Selector2 : Selector  NumberOfDimensions=2  IndexMode=Zero-based  IndexOptions=Index vector (port),Index vector (port)  Indices=0,[0:3]  OutputSizes=1,1
  Subtract : Sum  Inputs=+-
  Unary Minus : UnaryMinus
  SoftEndStopSt : Outport
  wires:
  Reshape1/1 -> EotDampgIncpt by VehSpd/3
  Reshape/1 -> EotEntrGainIncpt by VehSpd/3
  Selector1/1 -> Reshape/1
  Constant18/1 -> EotEntrGainIncpt by VehSpd/2
  Constant17/1 -> Selector1/1
  Constant16/1 -> EotDampgIncpt by VehSpd/2
  Selector2/1 -> Reshape1/1
  Constant15/1 -> Selector2/1
  Logical Operator5/1 -> If/4
  Logical Operator4/1 -> If/3
  Relational Operator3/1 -> Logical Operator5/2
  Relational Operator7/1 -> Logical Operator4/2, Logical Operator5/1
  Relational Operator2/1 -> Logical Operator4/1
  Constant14/1 -> Relational Operator7/2
  Data Store Read2/1 -> Relational Operator7/1
  Logical Operator3/1 -> If/2
  Logical Operator1/1 -> Logical Operator3/1
  Relational Operator4/1 -> Logical Operator3/2
  Relational Operator6/1 -> Logical Operator1/2
  Relational Operator5/1 -> Logical Operator1/1
  Constant12/1 -> Relational Operator6/2
  SysMotTqCmdSca/1 -> Relational Operator6/1
  Constant13/1 -> Relational Operator5/2
  Data Store Read1/1 -> Relational Operator5/1
  FixdToFloat_f32_u16/1 -> Subtract/2
  EotEntrGainIncpt by VehSpd/1 -> Max_u16/1
  End If/1 -> Data Store Write/1, SoftEndStopSt/1
  FloatToFixd_u16_f1/1 -> EotEntrGainIncpt by VehSpd/1
  EotDampgIncpt by VehSpd/1 -> Max_u16/2
  Data Store Read/1 -> Keep State/1(In1)
  FloatToFixd_u16_f32/1 -> EotDampgIncpt by VehSpd/1
  [VehSpd] -> FloatToFixd_u16_f32/1
  [VehSpd] -> FloatToFixd_u16_f1/1
  Max_u16/1 -> FixdToFloat_f32_u16/1
  Subtract/1 -> Relational Operator4/2
  Abslt_f32_f32/1 -> Subtract/1
  LimPosn/1 -> Abslt_f32_f32/1
  Abslt_f32_f1/1 -> Relational Operator4/1
  HwPosn/1 -> Abslt_f32_f1/1
  FildHwTq/1 -> Relational Operator3/1, Relational Operator2/1
  Keep State/1(Out1) -> End If/5
  PriorityVec2/1(Out1) -> End If/2
  PriorityVec4/1(Out1) -> End If/4
  If/2 -> PriorityVec2/Action  "StatePriVectRes"
  If/4 -> PriorityVec4/Action  "StatePriVectRes"
  If/3 -> PriorityVec3/Action  "StatePriVectRes"
  PriorityVec1/1(Out1) -> End If/1
  HwAuthy/1 -> Relational Operator/1
  Logical Operator2/1 -> Logical Operator/3
  Constant1/1 -> Relational Operator1/2
  Constant/1 -> Relational Operator/2
  Constant5/1 -> PriorityVec2/1(In1)
  Relational Operator1/1 -> Logical Operator/2
  EotDetd/1 -> Logical Operator2/1
  PriorityVec3/1(Out1) -> End If/3
  EotDi/1 -> Logical Operator/4
  Constant7/1 -> PriorityVec4/1(In1)
  Logical Operator/1 -> If/1
  VehSpd/1 -> [VehSpd]
  Relational Operator/1 -> Logical Operator/1
  Constant4/1 -> PriorityVec1/1(In1)
  If/1 -> PriorityVec1/Action  "StatePriVectRes"
  Constant6/1 -> PriorityVec3/1(In1)
  Constant2/1 -> Relational Operator2/2
  If/5 -> Keep State/Action
  [VehSpd] -> Relational Operator1/1
  Unary Minus/1 -> Relational Operator3/2
  Constant3/1 -> Unary Minus/1
  Constant8/1 -> Selector1/2
  Constant9/1 -> Selector1/3
  Constant10/1 -> Selector2/2
  Constant11/1 -> Selector2/3

== system SF018A_EotProtn/EotProtn/EotProtnPer1/EotDetd/CopyRight2 ==

== system SF018A_EotProtn/EotProtn/EotProtnPer1/EotVelImpct/CopyRight2 ==

== system SF018A_EotProtn/EotProtn/EotProtnPer1/EotVelImpct/If Action Subsystem ==
  In1 : Inport
  Action Port : ActionPort  ActionType=else
  CopyRight2 : Subsystem  Description=|  mask(Copyright Information){none=on}
      | Copyright info block.                                               
      |                                                                     
      | Place copyright information at the top of every subsystem in design.
      mask prompts: none "No parameters"
      mask help: Place copyright information at the top of every subsystem in design.
      mask Display:
      | NxtrConf = 'Nexteer Confidential';
      | 
      | sys = bdroot; %handle for the current model ("system")
      | first = get_param(sys,'Created');
      | if(isempty(first))
      |     first = datestr(now,'yyyy');
      | else
      |     first = first(end-3:end);  %year is last four digits
      | end
      | 
      | last = get_param(sys,'LastModifiedDate');
      | if isempty(last)
      |     last = datestr(now,'yyyy');
      | else
      |     last = last(end-3:end);
      | end
      | 
      | if strcmp(first,last)
      |     fprintf('%s -- Copyright %s Nexteer',NxtrConf,first)
      | else
      |     fprintf('%s -- %s%s- %s Nexteer',NxtrConf,char(169),first,last)
      | end
  Out1 : Outport
  wires:
  In1/1 -> Out1/1

== system SF018A_EotProtn/EotProtn/EotProtnPer1/EotVelImpct/If Action Subsystem1 ==
  In1 : Inport
  Action Port : ActionPort  ActionType=then
  CopyRight2 : Subsystem  Description=|  mask(Copyright Information){none=on}
      | Copyright info block.                                               
      |                                                                     
      | Place copyright information at the top of every subsystem in design.
      mask prompts: none "No parameters"
      mask help: Place copyright information at the top of every subsystem in design.
      mask Display:
      | NxtrConf = 'Nexteer Confidential';
      | 
      | sys = bdroot; %handle for the current model ("system")
      | first = get_param(sys,'Created');
      | if(isempty(first))
      |     first = datestr(now,'yyyy');
      | else
      |     first = first(end-3:end);  %year is last four digits
      | end
      | 
      | last = get_param(sys,'LastModifiedDate');
      | if isempty(last)
      |     last = datestr(now,'yyyy');
      | else
      |     last = last(end-3:end);
      | end
      | 
      | if strcmp(first,last)
      |     fprintf('%s -- Copyright %s Nexteer',NxtrConf,first)
      | else
      |     fprintf('%s -- %s%s- %s Nexteer',NxtrConf,char(169),first,last)
      | end
  Out1 : Outport
  wires:
  In1/1 -> Out1/1

== system SF018A_EotProtn/EotProtn/EotProtnPer1/EotVelImpct/If Action Subsystem2 ==
  In1 : Inport
  Action Port : ActionPort  ActionType=else
  CopyRight2 : Subsystem  Description=|  mask(Copyright Information){none=on}
      | Copyright info block.                                               
      |                                                                     
      | Place copyright information at the top of every subsystem in design.
      mask prompts: none "No parameters"
      mask help: Place copyright information at the top of every subsystem in design.
      mask Display:
      | NxtrConf = 'Nexteer Confidential';
      | 
      | sys = bdroot; %handle for the current model ("system")
      | first = get_param(sys,'Created');
      | if(isempty(first))
      |     first = datestr(now,'yyyy');
      | else
      |     first = first(end-3:end);  %year is last four digits
      | end
      | 
      | last = get_param(sys,'LastModifiedDate');
      | if isempty(last)
      |     last = datestr(now,'yyyy');
      | else
      |     last = last(end-3:end);
      | end
      | 
      | if strcmp(first,last)
      |     fprintf('%s -- Copyright %s Nexteer',NxtrConf,first)
      | else
      |     fprintf('%s -- %s%s- %s Nexteer',NxtrConf,char(169),first,last)
      | end
  Out1 : Outport
  wires:
  In1/1 -> Out1/1

== system SF018A_EotProtn/EotProtn/EotProtnPer1/EotVelImpct/If Action Subsystem3 ==
  In1 : Inport
  Action Port : ActionPort  ActionType=then
  CopyRight2 : Subsystem  Description=|  mask(Copyright Information){none=on}
      | Copyright info block.                                               
      |                                                                     
      | Place copyright information at the top of every subsystem in design.
      mask prompts: none "No parameters"
      mask help: Place copyright information at the top of every subsystem in design.
      mask Display:
      | NxtrConf = 'Nexteer Confidential';
      | 
      | sys = bdroot; %handle for the current model ("system")
      | first = get_param(sys,'Created');
      | if(isempty(first))
      |     first = datestr(now,'yyyy');
      | else
      |     first = first(end-3:end);  %year is last four digits
      | end
      | 
      | last = get_param(sys,'LastModifiedDate');
      | if isempty(last)
      |     last = datestr(now,'yyyy');
      | else
      |     last = last(end-3:end);
      | end
      | 
      | if strcmp(first,last)
      |     fprintf('%s -- Copyright %s Nexteer',NxtrConf,first)
      | else
      |     fprintf('%s -- %s%s- %s Nexteer',NxtrConf,char(169),first,last)
      | end
  Out1 : Outport
  wires:
  In1/1 -> Out1/1

== system SF018A_EotProtn/EotProtn/EotProtnPer1/EotVelImpct/If Action Subsystem4 ==
  In1 : Inport
  Action Port : ActionPort  ActionType=else
  CopyRight2 : Subsystem  Description=|  mask(Copyright Information){none=on}
      | Copyright info block.                                               
      |                                                                     
      | Place copyright information at the top of every subsystem in design.
      mask prompts: none "No parameters"
      mask help: Place copyright information at the top of every subsystem in design.
      mask Display:
      | NxtrConf = 'Nexteer Confidential';
      | 
      | sys = bdroot; %handle for the current model ("system")
      | first = get_param(sys,'Created');
      | if(isempty(first))
      |     first = datestr(now,'yyyy');
      | else
      |     first = first(end-3:end);  %year is last four digits
      | end
      | 
      | last = get_param(sys,'LastModifiedDate');
      | if isempty(last)
      |     last = datestr(now,'yyyy');
      | else
      |     last = last(end-3:end);
      | end
      | 
      | if strcmp(first,last)
      |     fprintf('%s -- Copyright %s Nexteer',NxtrConf,first)
      | else
      |     fprintf('%s -- %s%s- %s Nexteer',NxtrConf,char(169),first,last)
      | end
  Out1 : Outport
  wires:
  In1/1 -> Out1/1

== system SF018A_EotProtn/EotProtn/EotProtnPer1/EotVelImpct/If Action Subsystem5 ==
  In1 : Inport
  Action Port : ActionPort  ActionType=then
  CopyRight2 : Subsystem  Description=|  mask(Copyright Information){none=on}
      | Copyright info block.                                               
      |                                                                     
      | Place copyright information at the top of every subsystem in design.
      mask prompts: none "No parameters"
      mask help: Place copyright information at the top of every subsystem in design.
      mask Display:
      | NxtrConf = 'Nexteer Confidential';
      | 
      | sys = bdroot; %handle for the current model ("system")
      | first = get_param(sys,'Created');
      | if(isempty(first))
      |     first = datestr(now,'yyyy');
      | else
      |     first = first(end-3:end);  %year is last four digits
      | end
      | 
      | last = get_param(sys,'LastModifiedDate');
      | if isempty(last)
      |     last = datestr(now,'yyyy');
      | else
      |     last = last(end-3:end);
      | end
      | 
      | if strcmp(first,last)
      |     fprintf('%s -- Copyright %s Nexteer',NxtrConf,first)
      | else
      |     fprintf('%s -- %s%s- %s Nexteer',NxtrConf,char(169),first,last)
      | end
  Out1 : Outport
  wires:
  In1/1 -> Out1/1
